simulink model "BMS_MIL_Wrapper"  (R2025b)
settings: Solver=ode3  StartTime=0.0  StopTime=20  FixedStep=.001  RelTol=1e-3  EnableMultiTasking=on
InitFcn:
  | battery_init;
  | Full_Charge_Volt=4.2; % unit volts
  | Cutoff_Volt=3; % unit volts
  | Delta=.02;
  | ContactorTime=20;
  | ContactorTimeOut=100;
  | High_TempLim=333;
  | Low_TempLim=263;
  | Sensor_Fault_Treshold=.02;
  | CurrentTimeout=1;
  | Allowed_Delta=.04;
  | Bal_On_Time=30;
  | Bal_Off_Time=5;
  | BalNotAct_Time=10;
values from neighbouring files (symbols this model uses):
  bonka_R0 = [ ... (first row only)    [battery_init.m]
  bonka_SOC = [0, 0.1, 0.2, 0.3, 0.4, 0.5, 0.6, 0.7, 0.8, 0.9, 1.0]    [battery_init.m]
  bonka_T = [263.15, 273.15, 298.15, 313.15, 328.15]    [battery_init.m]
  Charge_Rate = 1    [battery_init.m]
  Discharge_Rate = -1    [battery_init.m]
  Fly_Cycle_Current = [ ... (first row only)    [battery_init.m]
undefined symbols (not defined in the file or in its folder): DiscIntNeverNeededParam, From_Plant_MATLABStruct, SRE
libraries: fl_lib x69, nesl_utility x54, simulink x35, ee_lib x12, batteryecm_lib x12, BatteryCurrentManagement x1
(part 2 of 4)

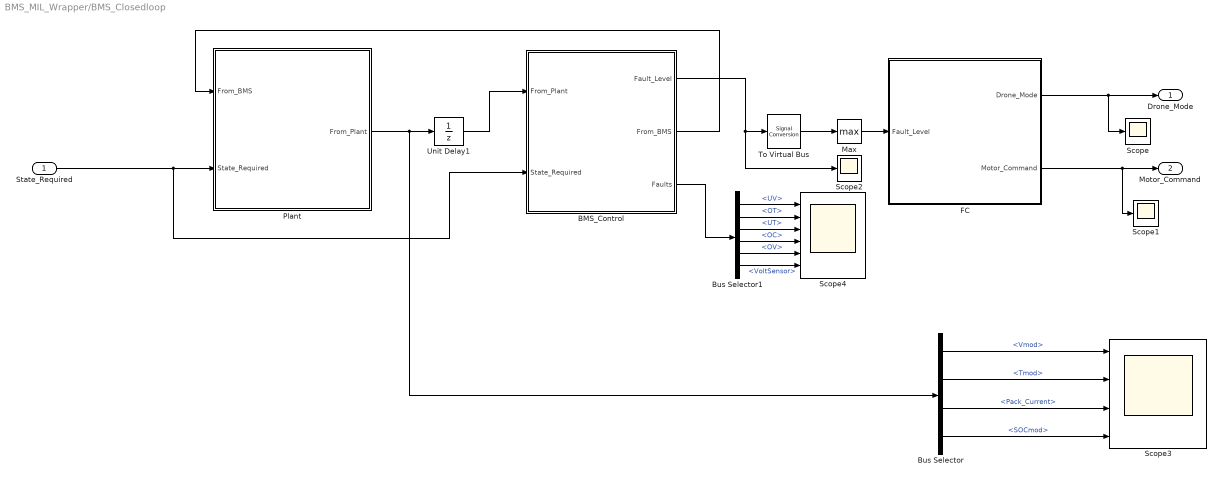
== system BMS_MIL_Wrapper/BMS_Closedloop ==
  State_Required : Inport
  BMS_Control : Subsystem
  Bus Selector : BusSelector  OutputSignals=Vmod,Tmod,Pack_Current,SOCmod
  Bus Selector1 : BusSelector  OutputSignals=UV,OT,UT,OC,OV,VoltSensor
  FC : Subsystem
  Max : MinMax  Function=max
  Plant : Subsystem
  Scope : Scope
      settings: ActiveDisplayYMinimum=-3.1634717321435111  ActiveDisplayYMaximum=3.4697725307175453  DataLoggingVariableName=ScopeData11
  Scope1 : Scope
      settings: ActiveDisplayYMinimum=-0.36691320387983084  ActiveDisplayYMaximum=1.2284387492451698  DataLoggingVariableName=ScopeData13
  Scope2 : Scope
      settings: ActiveDisplayYMinimum=-0.24999999999999994  ActiveDisplayYMaximum=2.25  DataLoggingVariableName=ScopeData14
  Scope3 : Scope  NumInputPorts=4
      settings: ActiveDisplayYMinimum=2.8974179415832806  ActiveDisplayYMaximum=3.7860858669734316
  Scope4 : Scope  NumInputPorts=6
      settings: ActiveDisplayYMinimum=-0.295339432217583  ActiveDisplayYMaximum=0.65647243137912314
  To Virtual Bus : SignalConversion  ConversionOutput=Virtual bus  OverrideOpt=off
  Unit Delay1 : UnitDelay  InitialCondition=From_Plant_MATLABStruct  SampleTime=-1  HasFrameUpgradeWarning=on
  Drone_Mode : Outport
  Motor_Command : Outport  Port=2
  wires:
  State_Required/1 -> BMS_Control/2(State_Required), Plant/2(State_Required)
  Plant/1(From_Plant) -> Unit Delay1/1, Bus Selector/1
  Unit Delay1/1 -> BMS_Control/1(From_Plant)
  Max/1 -> FC/1(Fault_Level)
  BMS_Control/1(Fault_Level) -> Scope2/1, To Virtual Bus/1
  FC/1(Drone_Mode) -> Scope/1, Drone_Mode/1
  FC/2(Motor_Command) -> Scope1/1, Motor_Command/1
  To Virtual Bus/1 -> Max/1
  BMS_Control/2(From_BMS) -> Plant/1(From_BMS)
  BMS_Control/3(Faults) -> Bus Selector1/1
  Bus Selector/1 -> Scope3/1  "<Vmod>"
  Bus Selector/2 -> Scope3/2  "<Tmod>"
  Bus Selector/3 -> Scope3/3  "<Pack_Current>"
  Bus Selector/4 -> Scope3/4  "<SOCmod>"
  Bus Selector1/5 -> Scope4/5  "<OV>"
  Bus Selector1/4 -> Scope4/4  "<OC>"
  Bus Selector1/3 -> Scope4/3  "<UT>"
  Bus Selector1/2 -> Scope4/2  "<OT>"
  Bus Selector1/1 -> Scope4/1  "<UV>"
  Bus Selector1/6 -> Scope4/6  "<VoltSensor>"

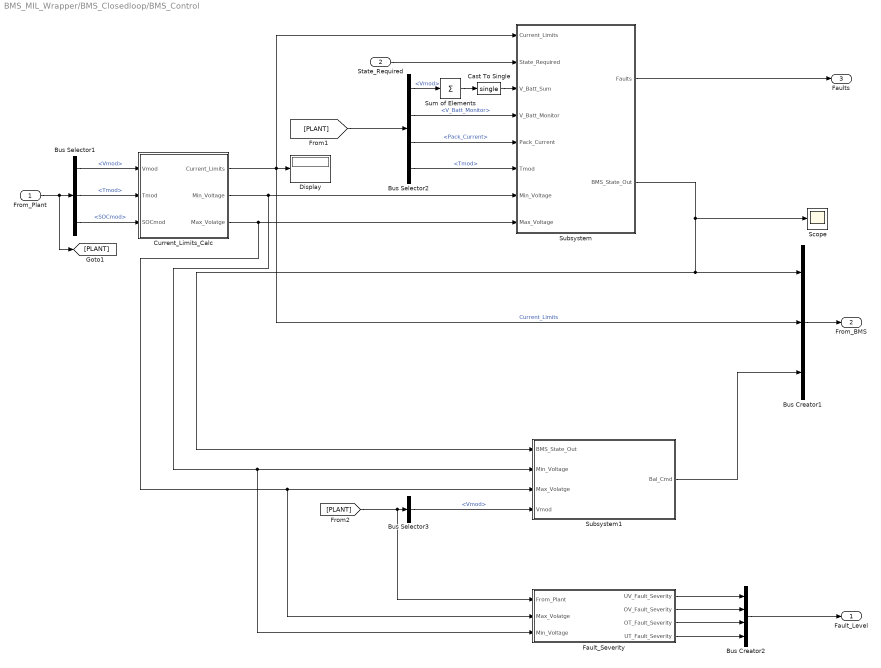
== system BMS_MIL_Wrapper/BMS_Closedloop/BMS_Control ==
  From_Plant : Inport
  State_Required : Inport  Port=2
  Bus Creator1 : BusCreator  Inputs=3
  Bus Creator2 : BusCreator  Inputs=4
  Bus Selector1 : BusSelector  OutputSignals=Vmod,Tmod,SOCmod
  Bus Selector2 : BusSelector  OutputSignals=Vmod,V_Batt_Monitor,Pack_Current,Tmod
  Bus Selector3 : BusSelector  OutputSignals=Vmod
  Cast To Single : DataTypeConversion  OutDataTypeStr=single  SaturateOnIntegerOverflow=off  RndMeth=Floor
  Current_Limits_Calc : Subsystem
  Display : Display
  Fault_Severity : Subsystem
  Scope : Scope
      settings: ActiveDisplayYMinimum=-1.5845803640246263  ActiveDisplayYMaximum=3.6127400845037951  DataLoggingVariableName=ScopeData3
  Subsystem : Subsystem
  Subsystem1 : Subsystem
  Sum of Elements : Sum  Inputs=+
  Fault_Level : Outport
  From_BMS : Outport  Port=2
  Faults : Outport  Port=3
  wires:
  From_Plant/1 -> [PLANT], Bus Selector1/1
  Bus Selector1/1 -> Current_Limits_Calc/1(Vmod)  "<Vmod>"
  Current_Limits_Calc/2(Min_Voltage) -> Fault_Severity/3(Min_Voltage), Subsystem1/2(Min_Voltage), Subsystem/7(Min_Voltage)
  Current_Limits_Calc/3(Max_Volatge) -> Subsystem/8(Max_Voltage), Fault_Severity/2(Max_Volatge), Subsystem1/3(Max_Volatge)
  Current_Limits_Calc/1(Current_Limits) -> Subsystem/1(Current_Limits), Bus Creator1/2, Display/1  "Current_Limits"
  State_Required/1 -> Subsystem/2(State_Required)
  [PLANT] -> Bus Selector2/1
  Subsystem/1(Faults) -> Faults/1
  Subsystem/2(BMS_State_Out) -> Scope/1, Bus Creator1/1, Subsystem1/1(BMS_State_Out)
  [PLANT] -> Fault_Severity/1(From_Plant), Bus Selector3/1
  Bus Selector3/1 -> Subsystem1/4(Vmod)  "<Vmod>"
  Subsystem1/1(Bal_Cmd) -> Bus Creator1/3
  Bus Selector2/1 -> Sum of Elements/1  "<Vmod>"
  Bus Selector2/4 -> Subsystem/6(Tmod)  "<Tmod>"
  Bus Selector2/2 -> Subsystem/4(V_Batt_Monitor)  "<V_Batt_Monitor>"
  Bus Selector2/3 -> Subsystem/5(Pack_Current)  "<Pack_Current>"
  Bus Selector1/2 -> Current_Limits_Calc/2(Tmod)  "<Tmod>"
  Bus Selector1/3 -> Current_Limits_Calc/3(SOCmod)  "<SOCmod>"
  Fault_Severity/4(UT_Fault_Severity) -> Bus Creator2/4
  Fault_Severity/3(OT_Fault_Severity) -> Bus Creator2/3
  Fault_Severity/2(OV_Fault_Severity) -> Bus Creator2/2
  Fault_Severity/1(UV_Fault_Severity) -> Bus Creator2/1
  Bus Creator2/1 -> Fault_Level/1
  Sum of Elements/1 -> Cast To Single/1
  Bus Creator1/1 -> From_BMS/1
  Cast To Single/1 -> Subsystem/3(V_Batt_Sum)

== system BMS_MIL_Wrapper/BMS_Closedloop/FC ==
  Fault_Level : Inport
  Chart : Stateflow chart  TreatAsAtomicUnit=on
  Drone_Mode : Outport
  Motor_Command : Outport  Port=2
  wires:
  Fault_Level/1 -> Chart/1(Fault_Level)
  Chart/1(Drone_Mode) -> Drone_Mode/1
  Chart/2(Motor_Command) -> Motor_Command/1

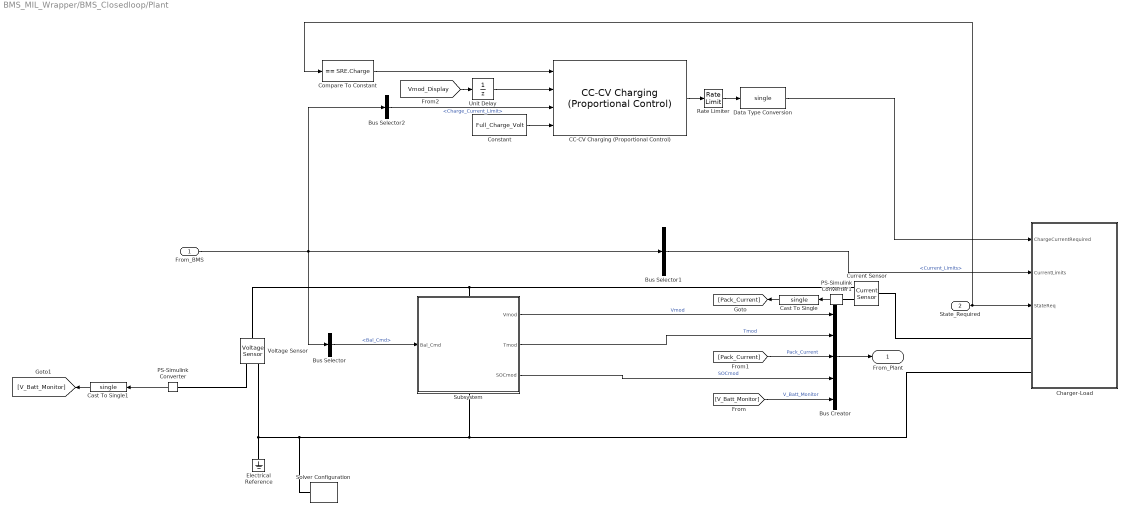
== system BMS_MIL_Wrapper/BMS_Closedloop/Plant ==
  From_BMS : Inport
  State_Required : Inport  Port=2
  Bus Creator : BusCreator  Inputs=5
  Bus Selector : BusSelector  OutputSignals=Bal_Cmd
  Bus Selector1 : BusSelector  OutputSignals=Current_Limits
  Bus Selector2 : BusSelector  OutputSignals=Current_Limits.Charge_Current_Limit
  CC-CV Charging (Proportional Control) : BatteryCurrentManagement/CC-CV Charging (Proportional Control)  MinMaxFlag=off  Kp=0.02  Ts=.001
      settings: LibrarySourceBlock=batt_sl_lib/Current Management/CC-CV Charging (Proportional Control)
  Cast To Single : DataTypeConversion  OutDataTypeStr=single  SaturateOnIntegerOverflow=off  RndMeth=Floor
  Cast To Single1 : DataTypeConversion  OutDataTypeStr=single  SaturateOnIntegerOverflow=off  RndMeth=Floor
  Charger-Load : Subsystem
  Compare To Constant : simulink/Logic and Bit Operations/Compare To Constant  relop===  const=SRE.Charge  OutDataTypeStr=boolean
  Constant : Constant  Value=Full_Charge_Volt
  Current Sensor : fl_lib/Electrical/Electrical Sensors/Current Sensor
  Data Type Conversion : DataTypeConversion  OutDataTypeStr=single  SaturateOnIntegerOverflow=off  RndMeth=Floor
  Electrical Reference : fl_lib/Electrical/Electrical Elements/Electrical Reference
  PS-Simulink Converter : nesl_utility/PS-Simulink Converter  PhysicalDomain=network_engine_domain  SubClassName=ps_output  LeftPortType=input  RightPortType=output  PseudoPeriodic=off  Frequencies=[]  VectorFormat=inherit  Unit=inherit  AffineConversion=off
  PS-Simulink Converter1 : nesl_utility/PS-Simulink Converter  PhysicalDomain=network_engine_domain  SubClassName=ps_output  LeftPortType=input  RightPortType=output  PseudoPeriodic=off  Frequencies=[]  VectorFormat=inherit  Unit=inherit  AffineConversion=off
  Rate Limiter : RateLimiter  RisingSlewLimit=10  FallingSlewLimit=-10  SampleTimeMode=inherited
  Solver Configuration : nesl_utility/Solver Configuration  PhysicalDomain=network_engine_domain  SubClassName=solver  LeftPortType=input  RightPortType=generic  Tones=[]  Harmonics=[]  SimulateNoise=off  Profile=off  UseLocalSampling=off  EnableSwitchedLinearOptims=on  FrequencyDomain=off  UseCCode=off  RelTol=0.001  AbsTol=0.001  MinStep=1e-09  ToWorkspace=off  RevertToSquareIcSolve=off  NumHomotopyIterations=100  PhasorMode=off  PhasorModeNumHarmonics=1  ConsistencySolver=NEWTON_XTOL_AFTER_FTOL  IndexReductionMethod=DerivativeReplacement  DoDC=off  ResidualTolerance=1e-09  ConsistencyTolSource=GLOBAL  ConsistencyAbsTol=0.001  ConsistencyRelTol=0.001  ConsistencyTolFactor=0.001  UseLocalSolver=on  LocalSolverChoice=NE_BACKWARD_EULER_ADVANCER  ResolveIndetEquations=on  FunctionEvalNumThread=1  LocalSolverSampleTime=0.001  DoFixedCost=off  MaxNonlinIter=3  MaxModeIter=2  ComputeImpulses=off  ImpulseIterations=2  LinearAlgebra=auto  LinearAlgebraNumThread=0  EquationFormulation=NE_TIME_EF  DelaysMemoryBudget=1024  AutomaticFiltering=on  FilteringTimeConstant=0.001  PartitionStorageMethod=AS_NEEDED  PartitionMemoryBudget=1024  PartitionMethod=ROBUST  MultibodyUseLocalSolver=off  MultibodyLocalSolverChoice=ODE1  MultibodyLocalSolverSampleTime=0.001
  Subsystem : Subsystem
      settings: PortSchema="{\"entries\":[{\"content\":{\"sides\":[{\"content\":{\"connectorIds\":[\"In1\"]},\"type\":\"ConnectorPlacement.EquallySpacedRectSide\",\"uuid\":\"58357de5-60ff-42e3-841b-e50425142caf\"},{\"content\":{\"connectorIds\":[\"Out1\",\"Out2\",\"Out3\"],\"side\":\"RIGHT\"},\"type\":\"ConnectorPlacement.EquallySpacedRectSide\",\"uuid\":\"e2d7d04f-a8ca-435a-9027-c1ea19fe7b57\"},{\"content\":{\"connectorIds\":[\"LConn1\"],\"side\":\"TOP\"},\"type\":\"ConnectorPlacement.EquallySpacedRectSide\",\"uuid\":\"61bcd3f6-6975-41f2-a4de-83d930262737\"},{\"content\":{\"connectorIds\":[\"RConn1\"],\"side\":\"BOTTOM\"},\"type\":\"ConnectorPlacement.EquallySpacedRectSide\",\"uuid\":\"f64ac1d4-74b0-46a5-b79a-ed01bae0794c\"}]},\"type\":\"ConnectorPlacement.EquallySpacedConnector\",\"uuid\":\"11abc81f-2488-49dd-a311-a0e5e9bbc669\"}],\"packageUris\":[\"http://schema.mathworks.com/mf0/Connector/R2020b\"],\"version\":\"1.0\"}"
  Unit Delay : UnitDelay  SampleTime=-1  HasFrameUpgradeWarning=on
  Voltage Sensor : fl_lib/Electrical/Electrical Sensors/Voltage Sensor
  From_Plant : Outport
  wires:
  Bus Creator/1 -> From_Plant/1
  Subsystem/1(Vmod) -> Bus Creator/1  "Vmod"
  Subsystem/2(Tmod) -> Bus Creator/2  "Tmod"
  PS-Simulink Converter/1 -> Cast To Single1/1
  [V_Batt_Monitor] -> Bus Creator/5  "V_Batt_Monitor"
  State_Required/1 -> Compare To Constant/1, Charger-Load/3(StateReq)
  Bus Selector1/1 -> Charger-Load/2(CurrentLimits)  "<Current_Limits>"
  Bus Selector/1 -> Subsystem/1(Bal_Cmd)  "<Bal_Cmd>"
  Subsystem/3(SOCmod) -> Bus Creator/4  "SOCmod"
  [Pack_Current] -> Bus Creator/3  "Pack_Current"
  Cast To Single/1 -> [Pack_Current]
  Cast To Single1/1 -> [V_Batt_Monitor]
  PS-Simulink Converter1/1 -> Cast To Single/1
  Bus Selector2/1 -> CC-CV Charging (Proportional Control)/3  "<Charge_Current_Limit>"
  Data Type Conversion/1 -> Charger-Load/1(ChargeCurrentRequired)
  Unit Delay/1 -> CC-CV Charging (Proportional Control)/2
  Constant/1 -> CC-CV Charging (Proportional Control)/4
  From_BMS/1 -> Bus Selector1/1, Bus Selector2/1, Bus Selector/1
  Compare To Constant/1 -> CC-CV Charging (Proportional Control)/1
  CC-CV Charging (Proportional Control)/1 -> Rate Limiter/1
  Rate Limiter/1 -> Data Type Conversion/1
  [Vmod_Display] -> Unit Delay/1
  connections:
  Subsystem/LConn1 -- Voltage Sensor/LConn1 -- Current Sensor/RConn2
  Voltage Sensor/RConn2 -- Electrical Reference/LConn1 -- Charger-Load/LConn2 -- Subsystem/RConn1 -- Solver Configuration/RConn1
  PS-Simulink Converter/LConn1 -- Voltage Sensor/RConn1
  Current Sensor/LConn1 -- Charger-Load/LConn1
  Current Sensor/RConn1 -- PS-Simulink Converter1/LConn1

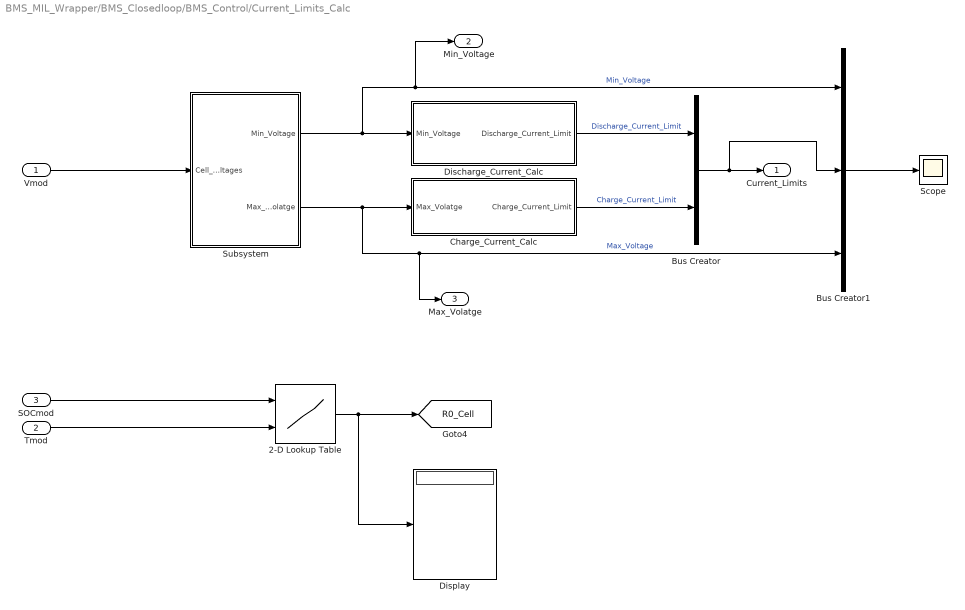
== system BMS_MIL_Wrapper/BMS_Closedloop/BMS_Control/Current_Limits_Calc ==
  Vmod : Inport
  Tmod : Inport  Port=2
  SOCmod : Inport  Port=3
  2-D Lookup Table : Lookup_n-D  BreakpointsForDimension1=bonka_SOC  BreakpointsForDimension2=bonka_T  Table=bonka_R0  InternalRulePriority=Speed  RndMeth=Simplest
      settings: InputPortMap=u0,u1
  Bus Creator : BusCreator  Inputs=2
  Bus Creator1 : BusCreator  Inputs=3
  Charge_Current_Calc : Subsystem
  Discharge_Current_Calc : Subsystem
  Display : Display
  Scope : Scope
      settings: ActiveDisplayYMinimum=-29.495145692080413  ActiveDisplayYMaximum=5.5081142916153993  DataLoggingVariableName=ScopeData2
  Subsystem : Subsystem
  Current_Limits : Outport
  Min_Voltage : Outport  Port=2
  Max_Volatge : Outport  Port=3
  tag scope: R0_Cell=global
  wires:
  Vmod/1 -> Subsystem/1(Cell_Voltages)
  Subsystem/1(Min_Voltage) -> Min_Voltage/1, Bus Creator1/1, Discharge_Current_Calc/1(Min_Voltage)  "Min_Voltage"
  Subsystem/2(Max_Volatge) -> Max_Volatge/1, Bus Creator1/3, Charge_Current_Calc/1(Max_Volatge)  "Max_Voltage"
  Discharge_Current_Calc/1(Discharge_Current_Limit) -> Bus Creator/1  "Discharge_Current_Limit"
  Charge_Current_Calc/1(Charge_Current_Limit) -> Bus Creator/2  "Charge_Current_Limit"
  Bus Creator/1 -> Bus Creator1/2, Current_Limits/1
  Bus Creator1/1 -> Scope/1
  2-D Lookup Table/1 -> Display/1, [R0_Cell]
  Tmod/1 -> 2-D Lookup Table/2
  SOCmod/1 -> 2-D Lookup Table/1

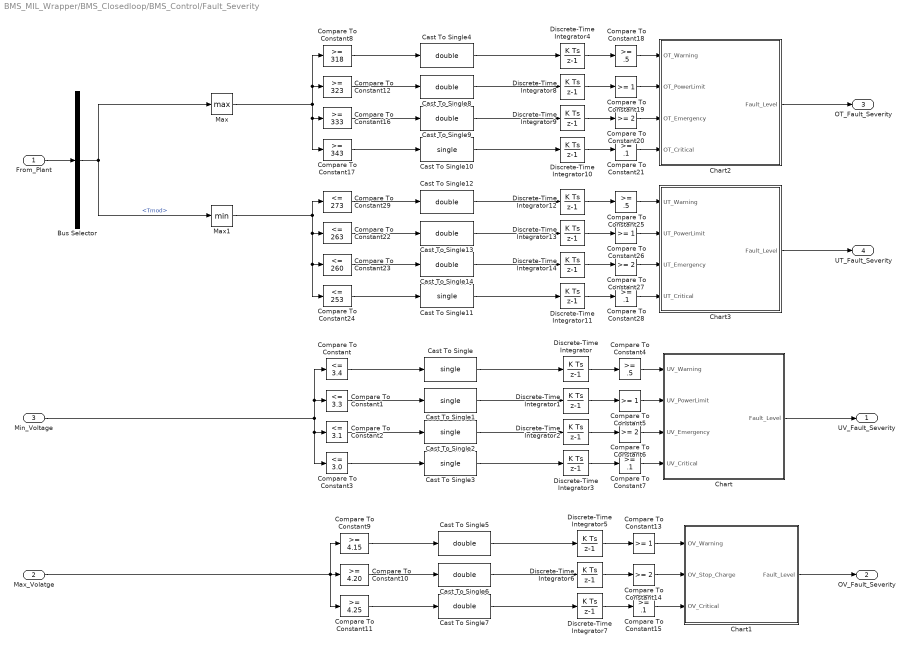
== system BMS_MIL_Wrapper/BMS_Closedloop/BMS_Control/Fault_Severity ==
  From_Plant : Inport
  Max_Volatge : Inport  Port=2
  Min_Voltage : Inport  Port=3
  Bus Selector : BusSelector  OutputSignals=Tmod
  Cast To Single{,1..3,10..11} (6 alike) : DataTypeConversion  OutDataTypeStr=single  SaturateOnIntegerOverflow=off  RndMeth=Floor
  Cast To Single{4..9,12..14} (9 alike) : DataTypeConversion  OutDataTypeStr=double  SaturateOnIntegerOverflow=off  RndMeth=Floor
  Chart : Stateflow chart  TreatAsAtomicUnit=on
  Chart1 : Stateflow chart  TreatAsAtomicUnit=on
  Chart2 : Stateflow chart  TreatAsAtomicUnit=on
  Chart3 : Stateflow chart  TreatAsAtomicUnit=on
  Compare To Constant : simulink/Logic and Bit Operations/Compare To Constant  relop=<=  const=3.4  OutDataTypeStr=boolean
  Compare To Constant1 : simulink/Logic and Bit Operations/Compare To Constant  relop=<=  const=3.3  OutDataTypeStr=boolean
  Compare To Constant10 : simulink/Logic and Bit Operations/Compare To Constant  relop=>=  const=4.20  OutDataTypeStr=boolean
  Compare To Constant11 : simulink/Logic and Bit Operations/Compare To Constant  relop=>=  const=4.25  OutDataTypeStr=boolean
  Compare To Constant12 : simulink/Logic and Bit Operations/Compare To Constant  relop=>=  const=323  OutDataTypeStr=boolean
  Compare To Constant{5,13,19,26} (4 alike) : simulink/Logic and Bit Operations/Compare To Constant  relop=>=  const=1  OutDataTypeStr=boolean
  Compare To Constant{6,14,20,27} (4 alike) : simulink/Logic and Bit Operations/Compare To Constant  relop=>=  const=2  OutDataTypeStr=boolean
  Compare To Constant{7,15,21,28} (4 alike) : simulink/Logic and Bit Operations/Compare To Constant  relop=>=  const=.1  OutDataTypeStr=boolean
  Compare To Constant16 : simulink/Logic and Bit Operations/Compare To Constant  relop=>=  const=333  OutDataTypeStr=boolean
  Compare To Constant17 : simulink/Logic and Bit Operations/Compare To Constant  relop=>=  const=343  OutDataTypeStr=boolean
  Compare To Constant18 : simulink/Logic and Bit Operations/Compare To Constant  relop=>=  const=.5  OutDataTypeStr=boolean
  Compare To Constant2 : simulink/Logic and Bit Operations/Compare To Constant  relop=<=  const=3.1  OutDataTypeStr=boolean
  Compare To Constant22 : simulink/Logic and Bit Operations/Compare To Constant  relop=<=  const=263  OutDataTypeStr=boolean
  Compare To Constant23 : simulink/Logic and Bit Operations/Compare To Constant  relop=<=  const=260  OutDataTypeStr=boolean
  Compare To Constant24 : simulink/Logic and Bit Operations/Compare To Constant  relop=<=  const=253  OutDataTypeStr=boolean
  Compare To Constant25 : simulink/Logic and Bit Operations/Compare To Constant  relop=>=  const=.5  OutDataTypeStr=boolean
  Compare To Constant29 : simulink/Logic and Bit Operations/Compare To Constant  relop=<=  const=273  OutDataTypeStr=boolean
  Compare To Constant3 : simulink/Logic and Bit Operations/Compare To Constant  relop=<=  const=3.0  OutDataTypeStr=boolean
  Compare To Constant4 : simulink/Logic and Bit Operations/Compare To Constant  relop=>=  const=.5  OutDataTypeStr=boolean
  Compare To Constant8 : simulink/Logic and Bit Operations/Compare To Constant  relop=>=  const=318  OutDataTypeStr=boolean
  Compare To Constant9 : simulink/Logic and Bit Operations/Compare To Constant  relop=>=  const=4.15  OutDataTypeStr=boolean
  Discrete-Time Integrator{,1..14} (15 alike) : DiscreteIntegrator  SampleTime=.001  ICPrevOutput=DiscIntNeverNeededParam  ICPrevScaledInput=DiscIntNeverNeededParam
  Max : MinMax  Function=max
  Max1 : MinMax
  UV_Fault_Severity : Outport
  OV_Fault_Severity : Outport  Port=2
  OT_Fault_Severity : Outport  Port=3
  UT_Fault_Severity : Outport  Port=4
  wires:
  From_Plant/1 -> Bus Selector/1
  Min_Voltage/1 -> Compare To Constant3/1, Compare To Constant2/1, Compare To Constant/1, Compare To Constant1/1
  Compare To Constant/1 -> Cast To Single/1
  Compare To Constant1/1 -> Cast To Single1/1
  Compare To Constant2/1 -> Cast To Single2/1
  Compare To Constant3/1 -> Cast To Single3/1
  Cast To Single/1 -> Discrete-Time Integrator/1
  Cast To Single1/1 -> Discrete-Time Integrator1/1
  Cast To Single2/1 -> Discrete-Time Integrator2/1
  Discrete-Time Integrator/1 -> Compare To Constant4/1
  Discrete-Time Integrator1/1 -> Compare To Constant5/1
  Discrete-Time Integrator2/1 -> Compare To Constant6/1
  Discrete-Time Integrator3/1 -> Compare To Constant7/1
  Cast To Single3/1 -> Discrete-Time Integrator3/1
  Compare To Constant4/1 -> Chart/1(UV_Warning)
  Compare To Constant5/1 -> Chart/2(UV_PowerLimit)
  Compare To Constant6/1 -> Chart/3(UV_Emergency)
  Compare To Constant7/1 -> Chart/4(UV_Critical)
  Chart/1(Fault_Level) -> UV_Fault_Severity/1
  Compare To Constant14/1 -> Chart1/2(OV_Stop_Charge)
  Max_Volatge/1 -> Compare To Constant9/1, Compare To Constant11/1, Compare To Constant10/1
  Discrete-Time Integrator6/1 -> Compare To Constant14/1
  Discrete-Time Integrator5/1 -> Compare To Constant13/1
  Compare To Constant13/1 -> Chart1/1(OV_Warning)
  Cast To Single6/1 -> Discrete-Time Integrator6/1
  Cast To Single7/1 -> Discrete-Time Integrator7/1
  Compare To Constant10/1 -> Cast To Single6/1
  Compare To Constant9/1 -> Cast To Single5/1
  Compare To Constant15/1 -> Chart1/3(OV_Critical)
  Compare To Constant11/1 -> Cast To Single7/1
  Chart1/1(Fault_Level) -> OV_Fault_Severity/1
  Discrete-Time Integrator7/1 -> Compare To Constant15/1
  Cast To Single5/1 -> Discrete-Time Integrator5/1
  Bus Selector/1 -> Max/1, Max1/1  "<Tmod>"
  Discrete-Time Integrator4/1 -> Compare To Constant18/1
  Compare To Constant20/1 -> Chart2/3(OT_Emergency)
  Max/1 -> Compare To Constant8/1, Compare To Constant12/1, Compare To Constant17/1, Compare To Constant16/1
  Discrete-Time Integrator9/1 -> Compare To Constant20/1
  Discrete-Time Integrator8/1 -> Compare To Constant19/1
  Compare To Constant19/1 -> Chart2/2(OT_PowerLimit)
  Cast To Single9/1 -> Discrete-Time Integrator9/1
  Cast To Single10/1 -> Discrete-Time Integrator10/1
  Cast To Single4/1 -> Discrete-Time Integrator4/1
  Compare To Constant16/1 -> Cast To Single9/1
  Compare To Constant12/1 -> Cast To Single8/1
  Compare To Constant21/1 -> Chart2/4(OT_Critical)
  Compare To Constant8/1 -> Cast To Single4/1
  Compare To Constant18/1 -> Chart2/1(OT_Warning)
  Compare To Constant17/1 -> Cast To Single10/1
  Chart2/1(Fault_Level) -> OT_Fault_Severity/1
  Discrete-Time Integrator10/1 -> Compare To Constant21/1
  Cast To Single8/1 -> Discrete-Time Integrator8/1
  Compare To Constant25/1 -> Chart3/1(UT_Warning)
  Max1/1 -> Compare To Constant22/1, Compare To Constant23/1, Compare To Constant24/1, Compare To Constant29/1
  Chart3/1(Fault_Level) -> UT_Fault_Severity/1
  Compare To Constant24/1 -> Cast To Single11/1
  Compare To Constant22/1 -> Cast To Single13/1
  Cast To Single13/1 -> Discrete-Time Integrator13/1
  Compare To Constant29/1 -> Cast To Single12/1
  Discrete-Time Integrator11/1 -> Compare To Constant28/1
  Compare To Constant23/1 -> Cast To Single14/1
  Discrete-Time Integrator14/1 -> Compare To Constant27/1
  Cast To Single14/1 -> Discrete-Time Integrator14/1
  Compare To Constant26/1 -> Chart3/2(UT_PowerLimit)
  Compare To Constant28/1 -> Chart3/4(UT_Critical)
  Cast To Single12/1 -> Discrete-Time Integrator12/1
  Discrete-Time Integrator13/1 -> Compare To Constant26/1
  Discrete-Time Integrator12/1 -> Compare To Constant25/1
  Compare To Constant27/1 -> Chart3/3(UT_Emergency)
  Cast To Single11/1 -> Discrete-Time Integrator11/1

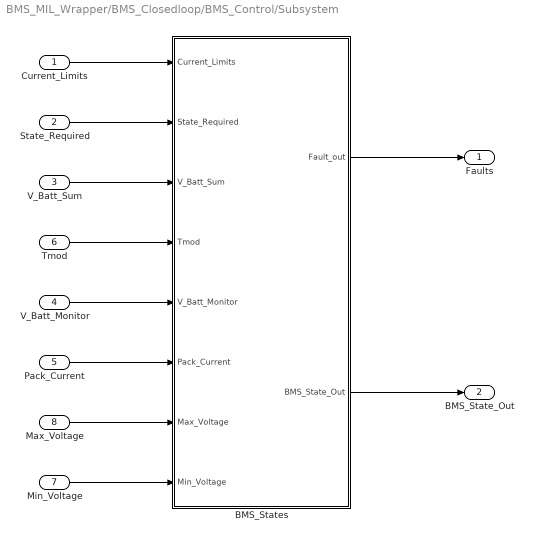
== system BMS_MIL_Wrapper/BMS_Closedloop/BMS_Control/Subsystem ==
  Current_Limits : Inport
  State_Required : Inport  Port=2
  V_Batt_Sum : Inport  Port=3
  V_Batt_Monitor : Inport  Port=4  OutDataTypeStr=single
  Pack_Current : Inport  Port=5  OutDataTypeStr=single
  Tmod : Inport  Port=6
  Min_Voltage : Inport  Port=7
  Max_Voltage : Inport  Port=8
  BMS_States : Stateflow chart  TreatAsAtomicUnit=on
      settings: PortSchema="{\"entries\":[{\"content\":{\"sides\":[{\"content\":{\"connectorIds\":[\"In1\",\"In6\",\"In3\",\"In2\",\"In5\",\"In4\",\"In7\",\"In8\"]},\"type\":\"ConnectorPlacement.EquallySpacedRectSide\",\"uuid\":\"75752650-a65f-4df2-8429-36d8f2b8ac99\"},{\"content\":{\"connectorIds\":[\"Out1\",\"Out2\"],\"side\":\"RIGHT\"},\"type\":\"ConnectorPlacement.EquallySpacedRectSide\",\"uuid\":\"5c64a1aa-fdb2-4c0c-b2ff-5c47ddc01ea2\"},{\"content\":{\"side\":\"TOP\"},\"type\":\"ConnectorPlacement.EquallySpacedRectSide\",\"uuid\":\"c92e07e0-a1c3-44d4-87a0-5a0cb4ce56f3\"}]},\"type\":\"ConnectorPlacement.EquallySpacedConnector\",\"uuid\":\"9d97857d-a16c-4ff3-995b-4c10703be4f7\"}],\"packageUris\":[\"http://schema.mathworks.com/mf0/Connector/R2020b\"],\"version\":\"1.0\"}"
  Faults : Outport
  BMS_State_Out : Outport  Port=2
  wires:
  Tmod/1 -> BMS_States/2(Tmod)
  Pack_Current/1 -> BMS_States/4(Pack_Current)
  V_Batt_Monitor/1 -> BMS_States/5(V_Batt_Monitor)
  Max_Voltage/1 -> BMS_States/7(Max_Voltage)
  Min_Voltage/1 -> BMS_States/8(Min_Voltage)
  State_Required/1 -> BMS_States/6(State_Required)
  Current_Limits/1 -> BMS_States/1(Current_Limits)
  BMS_States/1(Fault_out) -> Faults/1
  BMS_States/2(BMS_State_Out) -> BMS_State_Out/1
  V_Batt_Sum/1 -> BMS_States/3(V_Batt_Sum)

== system BMS_MIL_Wrapper/BMS_Closedloop/BMS_Control/Subsystem1 ==
  BMS_State_Out : Inport
  Min_Voltage : Inport  Port=2
  Max_Volatge : Inport  Port=3
  Vmod : Inport  Port=4
  Chart : Stateflow chart  TreatAsAtomicUnit=on
  Bal_Cmd : Outport
  wires:
  BMS_State_Out/1 -> Chart/1(BMS_State_Out)
  Min_Voltage/1 -> Chart/2(Min_Voltage)
  Chart/1(Bal_Cmd) -> Bal_Cmd/1
  Vmod/1 -> Chart/4(Vmod)
  Max_Volatge/1 -> Chart/3(Max_Voltage)

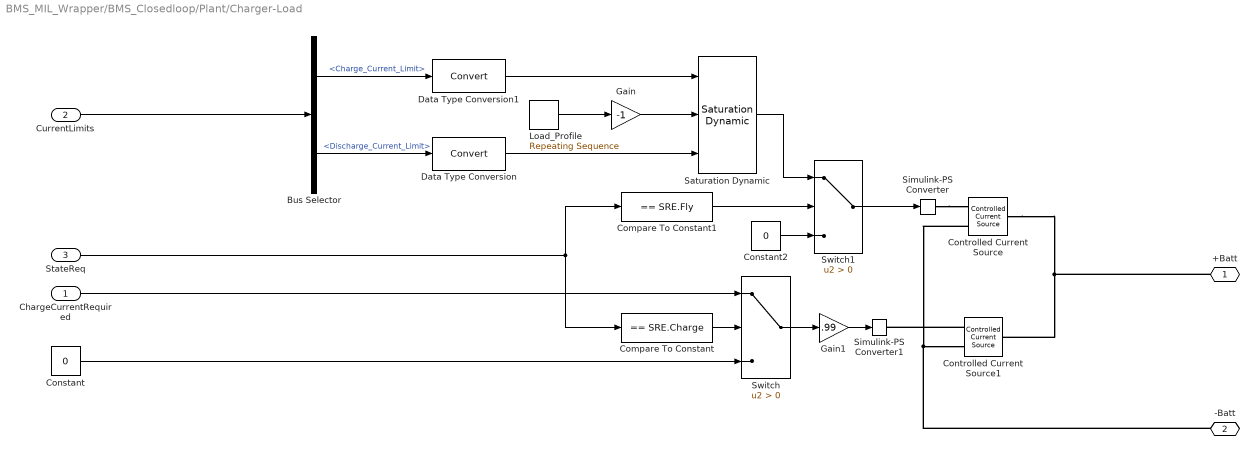
== system BMS_MIL_Wrapper/BMS_Closedloop/Plant/Charger-Load ==
  ChargeCurrentRequired : Inport
  CurrentLimits : Inport  Port=2
  StateReq : Inport  Port=3
  Bus Selector : BusSelector  OutputSignals=Charge_Current_Limit,Discharge_Current_Limit
  Compare To Constant : simulink/Logic and Bit Operations/Compare To Constant  relop===  const=SRE.Charge  OutDataTypeStr=boolean
  Compare To Constant1 : simulink/Logic and Bit Operations/Compare To Constant  relop===  const=SRE.Fly  OutDataTypeStr=boolean
  Constant : Constant  Value=0
  Constant2 : Constant  Value=0
  Controlled Current Source : fl_lib/Electrical/Electrical Sources/Controlled Current Source
  Controlled Current Source1 : fl_lib/Electrical/Electrical Sources/Controlled Current Source
  Data Type Conversion : DataTypeConversion  SaturateOnIntegerOverflow=off  RndMeth=Floor
  Data Type Conversion1 : DataTypeConversion  SaturateOnIntegerOverflow=off  RndMeth=Floor
  Gain : Gain  Gain=-1
  Gain1 : Gain  Gain=.99
  Load_Profile : simulink/Sources/Repeating Sequence  rep_seq_t=Fly_Cycle_Current (:,1)  rep_seq_y=Fly_Cycle_Current (:,2)
  Saturation Dynamic : simulink/Discontinuities/Saturation Dynamic  OutMin=[]  OutMax=[]  OutDataTypeStr=Inherit: Same as second input  OutDataType=fixdt(1, 16)  OutScaling=2^-10  DoSatur=off
  Simulink-PS Converter : nesl_utility/Simulink-PS Converter  PhysicalDomain=network_engine_domain  SubClassName=ps_input  LeftPortType=input  RightPortType=output  PseudoPeriodic=off  Frequencies=[]  NoiseDistribution=none  NoiseParameters=[]  Unit=1  AffineConversion=off  FilteringAndDerivatives=provide  SimscapeFilterOrder=1  InputFilterTimeConstant=0.001  UdotUserProvided=0
  Simulink-PS Converter1 : nesl_utility/Simulink-PS Converter  PhysicalDomain=network_engine_domain  SubClassName=ps_input  LeftPortType=input  RightPortType=output  PseudoPeriodic=off  Frequencies=[]  NoiseDistribution=none  NoiseParameters=[]  Unit=1  AffineConversion=off  FilteringAndDerivatives=provide  SimscapeFilterOrder=1  InputFilterTimeConstant=0.001  UdotUserProvided=0
  Switch : Switch  Criteria=u2 > Threshold  SaturateOnIntegerOverflow=off  InputSameDT=off
  Switch1 : Switch  Criteria=u2 > Threshold  SaturateOnIntegerOverflow=off  InputSameDT=off
  +Batt : PMIOPort  Side=Left
  -Batt : PMIOPort  Port=2  Side=Left
  wires:
  StateReq/1 -> Compare To Constant1/1, Compare To Constant/1
  Compare To Constant/1 -> Switch/2
  Switch/1 -> Gain1/1
  CurrentLimits/1 -> Bus Selector/1
  Gain/1 -> Saturation Dynamic/2
  Switch1/1 -> Simulink-PS Converter/1
  Saturation Dynamic/1 -> Switch1/1
  Compare To Constant1/1 -> Switch1/2
  Constant2/1 -> Switch1/3
  Bus Selector/1 -> Data Type Conversion1/1  "<Charge_Current_Limit>"
  Bus Selector/2 -> Data Type Conversion/1  "<Discharge_Current_Limit>"
  Data Type Conversion/1 -> Saturation Dynamic/3
  Data Type Conversion1/1 -> Saturation Dynamic/1
  Constant/1 -> Switch/3
  ChargeCurrentRequired/1 -> Switch/1
  Load_Profile/1 -> Gain/1
  Gain1/1 -> Simulink-PS Converter1/1
  connections:
  Simulink-PS Converter/RConn1 -- Controlled Current Source/RConn1
  Controlled Current Source1/RConn1 -- Simulink-PS Converter1/RConn1
  +Batt/RConn1 -- Controlled Current Source1/LConn1 -- Controlled Current Source/LConn1
  -Batt/RConn1 -- Controlled Current Source/RConn2 -- Controlled Current Source1/RConn2

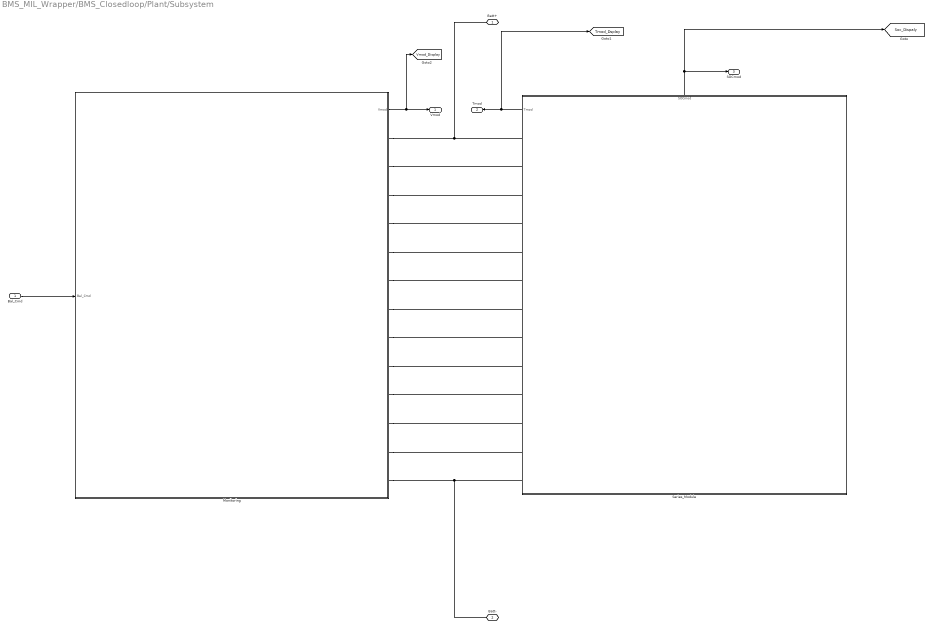
== system BMS_MIL_Wrapper/BMS_Closedloop/Plant/Subsystem ==
  Bal_Cmd : Inport  OutDataTypeStr=boolean
  Monitoring : Subsystem
  Series_Module : Subsystem
      settings: PortSchema="{\"entries\":[{\"content\":{\"sides\":[{\"content\":{\"connectorIds\":[\"Out2\",\"LConn1\",\"LConn2\",\"LConn3\",\"LConn4\",\"LConn5\",\"LConn6\",\"LConn7\",\"LConn8\",\"LConn9\",\"LConn10\",\"LConn11\",\"LConn12\",\"LConn13\"]},\"type\":\"ConnectorPlacement.EquallySpacedRectSide\",\"uuid\":\"c6d0ec2f-e215-49aa-88c4-aa36f54ff2d8\"},{\"content\":{\"side\":\"RIGHT\"},\"type\":\"ConnectorPlacement.EquallySpacedRectSide\",\"uuid\":\"ce965262-80da-4022-87ce-2d028a90e212\"},{\"content\":{\"connectorIds\":[\"Out1\"],\"side\":\"TOP\"},\"type\":\"ConnectorPlacement.EquallySpacedRectSide\",\"uuid\":\"06d9cb93-079f-49de-a983-b6840e947914\"}]},\"type\":\"ConnectorPlacement.EquallySpacedConnector\",\"uuid\":\"29985f6b-b161-490b-875e-190c720c1d7b\"}],\"packageUris\":[\"http://schema.mathworks.com/mf0/Connector/R2020b\"],\"version\":\"1.0\"}"
  Batt+ : PMIOPort  Side=Left
  Batt- : PMIOPort  Port=2  Side=Right
  Vmod : Outport
  Tmod : Outport  Port=2
  SOCmod : Outport  Port=3
  tag scope: Soc_Dispaly=global, Tmod_Dsplay=global, Vmod_Display=global
  wires:
  Bal_Cmd/1 -> Monitoring/1(Bal_Cmd)
  Monitoring/1(Vmod) -> [Vmod_Display], Vmod/1
  Series_Module/2(Tmod) -> [Tmod_Dsplay], Tmod/1
  Series_Module/1(SOCmod) -> [Soc_Dispaly], SOCmod/1
  connections:
  Monitoring/RConn1 -- Batt+/RConn1 -- Series_Module/LConn1
  Monitoring/RConn2 -- Series_Module/LConn2
  Monitoring/RConn3 -- Series_Module/LConn3
  Monitoring/RConn4 -- Series_Module/LConn4
  Monitoring/RConn5 -- Series_Module/LConn5
  Monitoring/RConn6 -- Series_Module/LConn6
  Monitoring/RConn7 -- Series_Module/LConn7
  Monitoring/RConn8 -- Series_Module/LConn8
  Monitoring/RConn9 -- Series_Module/LConn9
  Monitoring/RConn10 -- Series_Module/LConn10
  Monitoring/RConn11 -- Series_Module/LConn11
  Monitoring/RConn12 -- Series_Module/LConn12
  Monitoring/RConn13 -- Batt-/RConn1 -- Series_Module/LConn13

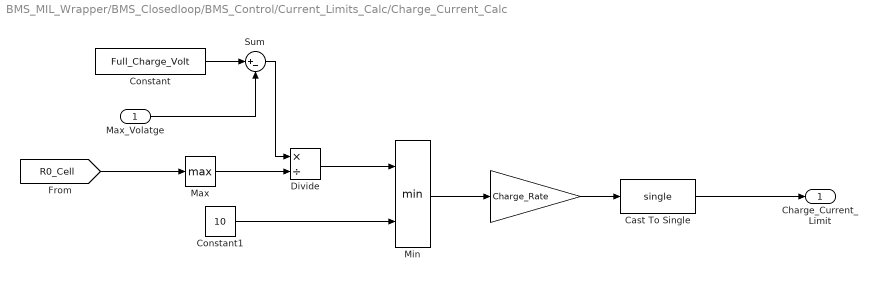
== system BMS_MIL_Wrapper/BMS_Closedloop/BMS_Control/Current_Limits_Calc/Charge_Current_Calc ==
  Max_Volatge : Inport
  " " : Gain  Gain=Charge_Rate
  Cast To Single : DataTypeConversion  OutDataTypeStr=single  SaturateOnIntegerOverflow=off  RndMeth=Floor
  Constant : Constant  Value=Full_Charge_Volt
  Constant1 : Constant  Value=10
  Divide : Product  Inputs=*/
  Max : MinMax  Function=max
  Min : MinMax  Inputs=2
  Sum : Sum  Inputs=|+-
  Charge_Current_Limit : Outport
  wires:
  Constant/1 -> Sum/1
  Max_Volatge/1 -> Sum/2
  Sum/1 -> Divide/1
  [R0_Cell] -> Max/1
  Divide/1 -> Min/1
  Cast To Single/1 -> Charge_Current_Limit/1
  " "/1 -> Cast To Single/1
  Max/1 -> Divide/2
  Min/1 -> " "/1
  Constant1/1 -> Min/2

== system BMS_MIL_Wrapper/BMS_Closedloop/BMS_Control/Current_Limits_Calc/Discharge_Current_Calc ==
  Min_Voltage : Inport
  Cast To Single : DataTypeConversion  OutDataTypeStr=single  SaturateOnIntegerOverflow=off  RndMeth=Floor
  Cutoff_Volt : Constant  Value=Cutoff_Volt
  Divide : Product  Inputs=*/
  Gain : Gain  Gain=Discharge_Rate
  Max : MinMax  Function=max
  Sum : Sum  Inputs=|+-
  Discharge_Current_Limit : Outport
  wires:
  Min_Voltage/1 -> Sum/1
  Cutoff_Volt/1 -> Sum/2
  Sum/1 -> Divide/1
  Max/1 -> Divide/2
  Divide/1 -> Gain/1
  Cast To Single/1 -> Discharge_Current_Limit/1
  Gain/1 -> Cast To Single/1
  [R0_Cell] -> Max/1

== system BMS_MIL_Wrapper/BMS_Closedloop/BMS_Control/Current_Limits_Calc/Subsystem ==
  Cell_Voltages : Inport
  Max : MinMax  Function=max
  MinMax : MinMax
  Min_Voltage : Outport
  Max_Volatge : Outport  Port=2
  wires:
  Cell_Voltages/1 -> Max/1, MinMax/1
  MinMax/1 -> Min_Voltage/1
  Max/1 -> Max_Volatge/1

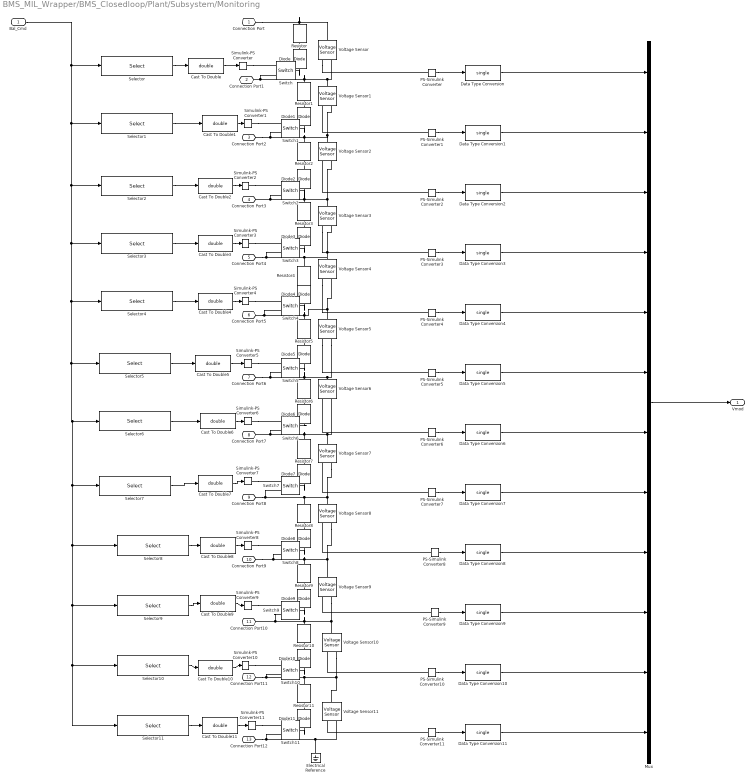
== system BMS_MIL_Wrapper/BMS_Closedloop/Plant/Subsystem/Monitoring ==
  Bal_Cmd : Inport  OutDataTypeStr=boolean
  Cast To Double{,1..11} (12 alike) : DataTypeConversion  OutDataTypeStr=double  SaturateOnIntegerOverflow=off  RndMeth=Floor
  Data Type Conversion{,1..11} (12 alike) : DataTypeConversion  OutDataTypeStr=single  SaturateOnIntegerOverflow=off  RndMeth=Floor
  Diode{,1..11} (12 alike) : ee_lib/Semiconductors & Converters/Diode  ModelType=ee.enum.diode.modelType.pwl  TableType=ee.enum.diode.tableType.IfMat  IfMat=[.07, .12, .19, 1.75, 4.24, 7.32, 11.2; .16, .3, .72, 2.14, 5.02, 8.35, 13.12] A  VfMat=[.9, 1.15, 1.25, 1.5, 1.75, 2.17, 2.6, 2.85; .58, .68, .75, 1.1, 1.38, 1.77, 2.27, 2.7] V  TjVec=[25, 125] degC  VfVec=[.5, .7, .9, 1.3, 1.7, 2.1, 2.5] V  IfVec=[.1, .2, .5, 1, 2, 4, 7, 10] A  IrMat=[1e-06, 2e-06, 5e-06, 1e-05, 2.5e-05, 5e-05, .0001; 2e-06, 5e-06, 1e-05, 4e-05, 8e-05, .0002, .0005] A  VrMat=[10, 100, 200, 250, 300, 325, 350; 10, 70, 160, 220, 270, 300, 320] V  VrVec=[10, 20, 40, 50, 70, 80, 100] V  IrVec=[1e-06, 2e-06, 5e-06, 1e-05, 2e-05, 5e-05, .0001] A  Vf=0.6 V  Ron=0.3 Ohm  Goff=1e-8 S  prmExp=ee.enum.diode.expParam.useTwo  I12=[.0137, .545] A  V12=[.6, .7] V  RS=0 Ohm  Tmeas=298.15 K  IS=1e-12 A  ec=1  I1=0.0137 A  V1=0.6 V  N_series=1  N_parallel=1  ZenerEnable=false  Rz=0.3 Ohm  BV=inf V  C_param=ee.enum.diode.capParam.fixed  CJ=0 pF  CJ0=5 pF  Vvec=[.1, 10, 100] V  Cvec=[3.5, 1, .4] pF  VJ=1 V  Mgrad=0.5  FC=0.5  Q_param=ee.enum.diode.recoveryParam.off  iRM=-7.15 A  iF=4 A  didt=-750 A/us  trr_factor=3  trr=115 ns  Qrr=150 nA*s  Vr=-600 V  Ls=150 nH  Erec=0.03 J  TT=50 ns  tau=100 ns  T_param=ee.enum.diode.temperatureParam.off  Tdevice=298.15 K  I1_T2=0.245 A  V1_T2=0.5 V  IS_T2=1.25e-7 A  Tmeas2=125 degC  XTI_param=ee.enum.diode.xtiParam.pn  XTI=3  EG_param=ee.enum.diode.egapParam.material_si  EG=1.11 eV  dBVdT=0 V/K  enable_fault_input=simscape.enum.onoff.off  i_specify=off  i_priority=None  i=0 A  i_nominal_specify=off  i_nominal_value=1  i_nominal_unit=A  v_specify=off  v_priority=None  v=0 V  v_nominal_specify=off  v_nominal_value=1  v_nominal_unit=V  v_capacitor_specify=off  v_capacitor_priority=None  v_capacitor=0 V  v_capacitor_nominal_specify=off  v_capacitor_nominal_value=1  v_capacitor_nominal_unit=V  Qj_specify=off  Qj_priority=High  Qj=0 C  Qj_nominal_specify=off  Qj_nominal_value=1  Qj_nominal_unit=C  i_diode_specify=off  i_diode_priority=None  i_diode=0 A  i_diode_nominal_specify=off  i_diode_nominal_value=1  i_diode_nominal_unit=A  v_diode_specify=off  v_diode_priority=None  v_diode=0 V  v_diode_nominal_specify=off  v_diode_nominal_value=1  v_diode_nominal_unit=V  i_capacitor_specify=off  i_capacitor_priority=None  i_capacitor=0 A  i_capacitor_nominal_specify=off  i_capacitor_nominal_value=1  i_capacitor_nominal_unit=A  power_dissipated_specify=off  power_dissipated_priority=None  power_dissipated=0 W  power_dissipated_nominal_specify=off  power_dissipated_nominal_value=1  power_dissipated_nominal_unit=W  fidelity_level=ee.enum.diode.fidelity.includeChargeDyn  rec_loss_model=ee.enum.diode.reverseRecoveryModel.fixed  ErecVal=0 J  scaleWithIandV=true  ErecMat=zeros(2, 3) J  TjrecVec=[298.15, 398.15] K  IfrecVec=[.1, 1, 10] A  IrecVal=10 A  VrecVal=10 V  tFilter=1 / 1000 / 100 s  thermal_network_parameterization=ee.enum.thermalNetworkTopology.junctionCase  Rth=[0, 10] K/W  Rth_Cauer=[1, 3, 10] K/W  Rth_Foster=[.08, .14, .22, .16] K/W  thermal_mass_parameterization=ee.enum.thermalNetwork.timeconstant  thermal_mass=[0, 1] J/K  thermal_mass_Cauer=[.1, .3, 1] J/K  thermal_mass_Foster=[.001, .005, .05, .5] J/K  thermal_time_constant=[0, 10] s  thermal_time_constant_Cauer=[1, 3, 10] s  thermal_time_constant_Foster=[7e-05, .0007, .01, .08] s  thermal_mass_initial_temperatures=[25, 25] degC  thermal_mass_initial_temperatures_Cauer=[25, 25, 25] degC  junction_thermal_mass=0.01 J/K  Tvec_initial_Foster=[25, 25, 25, 25] degC  no_thermal_network=0  junction_temperature_specify=off  junction_temperature_priority=None  junction_temperature=25 degC  junction_temperature_nominal_specify=off  junction_temperature_nominal_value=1  junction_temperature_nominal_unit=degC
  Electrical Reference : fl_lib/Electrical/Electrical Elements/Electrical Reference
  Mux : Mux  Inputs=12
  PS-Simulink Converter{,1..11} (12 alike) : nesl_utility/PS-Simulink Converter  PhysicalDomain=network_engine_domain  SubClassName=ps_output  LeftPortType=input  RightPortType=output  PseudoPeriodic=off  Frequencies=[]  VectorFormat=inherit  Unit=inherit  AffineConversion=off
  Resistor{,1..11} (12 alike) : fl_lib/Electrical/Electrical Elements/Resistor  R=39 Ohm  i_specify=off  i_priority=None  i=0 A  i_nominal_specify=off  i_nominal_value=1  i_nominal_unit=A  v_specify=off  v_priority=None  v=0 V  v_nominal_specify=off  v_nominal_value=1  v_nominal_unit=V
  Selector : Selector  InputPortWidth=12  IndexOptions=Index vector (dialog)  Indices=1  OutputSizes=1
  Selector1 : Selector  InputPortWidth=12  IndexOptions=Index vector (dialog)  Indices=2  OutputSizes=1
  Selector10 : Selector  InputPortWidth=12  IndexOptions=Index vector (dialog)  Indices=11  OutputSizes=1
  Selector11 : Selector  InputPortWidth=12  IndexOptions=Index vector (dialog)  Indices=12  OutputSizes=1
  Selector2 : Selector  InputPortWidth=12  IndexOptions=Index vector (dialog)  Indices=3  OutputSizes=1
  Selector3 : Selector  InputPortWidth=12  IndexOptions=Index vector (dialog)  Indices=4  OutputSizes=1
  Selector4 : Selector  InputPortWidth=12  IndexOptions=Index vector (dialog)  Indices=5  OutputSizes=1
  Selector5 : Selector  InputPortWidth=12  IndexOptions=Index vector (dialog)  Indices=6  OutputSizes=1
  Selector6 : Selector  InputPortWidth=12  IndexOptions=Index vector (dialog)  Indices=7  OutputSizes=1
  Selector7 : Selector  InputPortWidth=12  IndexOptions=Index vector (dialog)  Indices=8  OutputSizes=1
  Selector8 : Selector  InputPortWidth=12  IndexOptions=Index vector (dialog)  Indices=9  OutputSizes=1
  Selector9 : Selector  InputPortWidth=12  IndexOptions=Index vector (dialog)  Indices=10  OutputSizes=1
  Simulink-PS Converter{,1..11} (12 alike) : nesl_utility/Simulink-PS Converter  PhysicalDomain=network_engine_domain  SubClassName=ps_input  LeftPortType=input  RightPortType=output  PseudoPeriodic=off  Frequencies=[]  NoiseDistribution=none  NoiseParameters=[]  Unit=1  AffineConversion=off  FilteringAndDerivatives=provide  SimscapeFilterOrder=1  InputFilterTimeConstant=0.001  UdotUserProvided=0
  Switch{,1..11} (12 alike) : fl_lib/Electrical/Electrical Elements/Switch  R_closed=0.01 Ohm  G_open=1e-8 1/Ohm  Threshold=0.5  i_specify=off  i_priority=None  i=0 A  i_nominal_specify=off  i_nominal_value=1  i_nominal_unit=A  v_specify=off  v_priority=None  v=0 V  v_nominal_specify=off  v_nominal_value=1  v_nominal_unit=V
  Voltage Sensor{,1..11} (12 alike) : fl_lib/Electrical/Electrical Sensors/Voltage Sensor
  Connection Port : PMIOPort  Side=Right
  Connection Port1 : PMIOPort  Port=2  Side=Right
  Connection Port2 : PMIOPort  Port=3  Side=Right
  Connection Port3 : PMIOPort  Port=4  Side=Right
  Connection Port4 : PMIOPort  Port=5  Side=Right
  Connection Port5 : PMIOPort  Port=6  Side=Right
  Connection Port6 : PMIOPort  Port=7  Side=Right
  Connection Port7 : PMIOPort  Port=8  Side=Right
  Connection Port8 : PMIOPort  Port=9  Side=Right
  Connection Port9 : PMIOPort  Port=10  Side=Right
  Connection Port10 : PMIOPort  Port=11  Side=Right
  Connection Port11 : PMIOPort  Port=12  Side=Right
  Connection Port12 : PMIOPort  Port=13  Side=Right
  Vmod : Outport
  wires:
  PS-Simulink Converter/1 -> Data Type Conversion/1
  PS-Simulink Converter1/1 -> Data Type Conversion1/1
  PS-Simulink Converter2/1 -> Data Type Conversion2/1
  PS-Simulink Converter3/1 -> Data Type Conversion3/1
  PS-Simulink Converter4/1 -> Data Type Conversion4/1
  PS-Simulink Converter5/1 -> Data Type Conversion5/1
  PS-Simulink Converter6/1 -> Data Type Conversion6/1
  PS-Simulink Converter7/1 -> Data Type Conversion7/1
  PS-Simulink Converter8/1 -> Data Type Conversion8/1
  PS-Simulink Converter9/1 -> Data Type Conversion9/1
  PS-Simulink Converter10/1 -> Data Type Conversion10/1
  PS-Simulink Converter11/1 -> Data Type Conversion11/1
  Data Type Conversion/1 -> Mux/1
  Data Type Conversion1/1 -> Mux/2
  Data Type Conversion2/1 -> Mux/3
  Data Type Conversion3/1 -> Mux/4
  Data Type Conversion4/1 -> Mux/5
  Data Type Conversion5/1 -> Mux/6
  Data Type Conversion6/1 -> Mux/7
  Data Type Conversion7/1 -> Mux/8
  Data Type Conversion8/1 -> Mux/9
  Data Type Conversion9/1 -> Mux/10
  Data Type Conversion10/1 -> Mux/11
  Data Type Conversion11/1 -> Mux/12
  Bal_Cmd/1 -> Selector/1, Selector2/1, Selector3/1, Selector4/1, Selector5/1, Selector10/1, Selector11/1, Selector9/1, Selector8/1, Selector7/1, Selector6/1, Selector1/1
  Mux/1 -> Vmod/1
  Selector/1 -> Cast To Double/1
  Cast To Double/1 -> Simulink-PS Converter/1
  Cast To Double1/1 -> Simulink-PS Converter1/1
  Selector1/1 -> Cast To Double1/1
  Selector2/1 -> Cast To Double2/1
  Cast To Double2/1 -> Simulink-PS Converter2/1
  Selector3/1 -> Cast To Double3/1
  Cast To Double3/1 -> Simulink-PS Converter3/1
  Selector4/1 -> Cast To Double4/1
  Cast To Double4/1 -> Simulink-PS Converter4/1
  Selector5/1 -> Cast To Double5/1
  Cast To Double5/1 -> Simulink-PS Converter5/1
  Selector6/1 -> Cast To Double6/1
  Cast To Double6/1 -> Simulink-PS Converter6/1
  Cast To Double7/1 -> Simulink-PS Converter7/1
  Selector7/1 -> Cast To Double7/1
  Selector8/1 -> Cast To Double8/1
  Cast To Double8/1 -> Simulink-PS Converter8/1
  Selector9/1 -> Cast To Double9/1
  Cast To Double9/1 -> Simulink-PS Converter9/1
  Cast To Double10/1 -> Simulink-PS Converter10/1
  Selector10/1 -> Cast To Double10/1
  Cast To Double11/1 -> Simulink-PS Converter11/1
  Selector11/1 -> Cast To Double11/1
  connections:
  Connection Port/RConn1 -- Voltage Sensor/LConn1 -- Resistor/LConn1
  Connection Port1/RConn1 -- Switch/RConn2 -- Resistor1/LConn1 -- Voltage Sensor/RConn2 -- Voltage Sensor1/LConn1
  Connection Port2/RConn1 -- Voltage Sensor1/RConn2 -- Voltage Sensor2/LConn1 -- Resistor2/LConn1 -- Switch1/RConn2
  Connection Port4/RConn1 -- Switch3/RConn2 -- Resistor4/LConn1 -- Voltage Sensor4/LConn1 -- Voltage Sensor3/RConn2
  Connection Port5/RConn1 -- Switch4/RConn2 -- Resistor5/LConn1 -- Voltage Sensor4/RConn2 -- Voltage Sensor5/LConn1
  Voltage Sensor7/LConn1 -- Voltage Sensor6/RConn2 -- Resistor7/LConn1 -- Switch6/RConn2 -- Connection Port7/RConn1
  Voltage Sensor7/RConn2 -- Resistor8/LConn1 -- Switch7/RConn2 -- Connection Port8/RConn1 -- Voltage Sensor8/LConn1
  Connection Port12/RConn1 -- Switch11/RConn2 -- Electrical Reference/LConn1 -- Voltage Sensor11/RConn2
  Voltage Sensor/RConn1 -- PS-Simulink Converter/LConn1
  PS-Simulink Converter1/LConn1 -- Voltage Sensor1/RConn1
  PS-Simulink Converter2/LConn1 -- Voltage Sensor2/RConn1
  Voltage Sensor3/RConn1 -- PS-Simulink Converter3/LConn1
  Voltage Sensor4/RConn1 -- PS-Simulink Converter4/LConn1
  Voltage Sensor5/RConn1 -- PS-Simulink Converter5/LConn1
  PS-Simulink Converter6/LConn1 -- Voltage Sensor6/RConn1
  PS-Simulink Converter7/LConn1 -- Voltage Sensor7/RConn1
  PS-Simulink Converter8/LConn1 -- Voltage Sensor8/RConn1
  PS-Simulink Converter9/LConn1 -- Voltage Sensor9/RConn1
  PS-Simulink Converter10/LConn1 -- Voltage Sensor10/RConn1
  PS-Simulink Converter11/LConn1 -- Voltage Sensor11/RConn1
  Diode/LConn1 -- Resistor/RConn1
  Diode/RConn1 -- Switch/LConn1
  Resistor1/RConn1 -- Diode1/LConn1
  Diode1/RConn1 -- Switch1/LConn1
  Diode2/RConn1 -- Switch2/LConn1
  Voltage Sensor3/LConn1 -- Resistor3/LConn1 -- Switch2/RConn2 -- Connection Port3/RConn1 -- Voltage Sensor2/RConn2
  Resistor3/RConn1 -- Diode3/LConn1
  Diode3/RConn1 -- Switch3/LConn1
  Resistor4/RConn1 -- Diode4/LConn1
  Diode4/RConn1 -- Switch4/LConn1
  Voltage Sensor5/RConn2 -- Resistor6/LConn1 -- Switch5/RConn2 -- Connection Port6/RConn1 -- Voltage Sensor6/LConn1
  Resistor5/RConn1 -- Diode5/LConn1
  Diode5/RConn1 -- Switch5/LConn1
  Resistor6/RConn1 -- Diode6/LConn1
  Switch6/LConn1 -- Diode6/RConn1
  Resistor7/RConn1 -- Diode7/LConn1
  Diode7/RConn1 -- Switch7/LConn1
  Voltage Sensor8/RConn2 -- Resistor9/LConn1 -- Switch8/RConn2 -- Connection Port9/RConn1 -- Voltage Sensor9/LConn1
  Resistor8/RConn1 -- Diode8/LConn1
  Diode8/RConn1 -- Switch8/LConn1
  Voltage Sensor9/RConn2 -- Voltage Sensor10/LConn1 -- Resistor10/LConn1 -- Switch9/RConn2 -- Connection Port10/RConn1
  Resistor9/RConn1 -- Diode9/LConn1
  Diode9/RConn1 -- Switch9/LConn1
  Voltage Sensor10/RConn2 -- Resistor11/LConn1 -- Switch10/RConn2 -- Connection Port11/RConn1 -- Voltage Sensor11/LConn1
  Resistor10/RConn1 -- Diode10/LConn1
  Diode10/RConn1 -- Switch10/LConn1
  Diode11/RConn1 -- Switch11/LConn1
  Diode11/LConn1 -- Resistor11/RConn1
  Simulink-PS Converter/RConn1 -- Switch/RConn1
  Simulink-PS Converter1/RConn1 -- Switch1/RConn1
  Simulink-PS Converter2/RConn1 -- Switch2/RConn1
  Simulink-PS Converter3/RConn1 -- Switch3/RConn1
  Simulink-PS Converter11/RConn1 -- Switch11/RConn1
  Simulink-PS Converter10/RConn1 -- Switch10/RConn1
  Simulink-PS Converter9/RConn1 -- Switch9/RConn1
  Simulink-PS Converter8/RConn1 -- Switch8/RConn1
  Simulink-PS Converter7/RConn1 -- Switch7/RConn1
  Simulink-PS Converter6/RConn1 -- Switch6/RConn1
  Simulink-PS Converter5/RConn1 -- Switch5/RConn1
  Simulink-PS Converter4/RConn1 -- Switch4/RConn1
  Diode2/LConn1 -- Resistor2/RConn1
